simulink model "ampc_pH_lpv"  (R2021a)
settings: Solver=ode45  StartTime=0.0  StopTime=100  MaxStep=0.1  RelTol=1e-3
undefined symbols (not defined in the file or in its folder): sigbuilder_block
libraries: mpclib x1, cstblocks x1, simulink x1
settings Model: Creator=Oluwatofunmi  LastModifiedBy=USER
settings SolverCC: ZeroCrossAlgorithm=Adaptive  AlgebraicLoopSolver=TrustRegion
settings DebuggingCC: PregeneratedLibrarySubsystemCodeDiagnostic=none  SFMachineParentedDataDiag=warning  ArithmeticOperatorsInVariantConditions=warning
settings SFSimCC: CustomCodeUndefinedFunction=UseInterfaceOnly

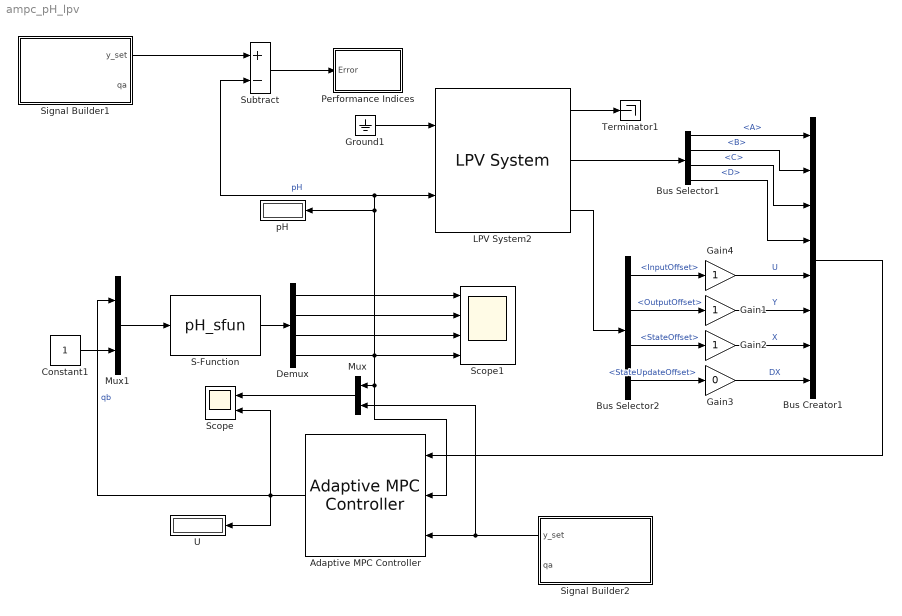
== system ampc_pH_lpv ==
  Adaptive MPC Controller : mpclib/Adaptive MPC Controller  SCDEnableBlockLinearizationSpecification=on  mpcobj=mpcobj_lpv  enable_value=0  updateMPCinCallerWorkspace=on  md_inport=off  mv_inport=off  uref_inport=off  return_cost=off  return_mvseq=off  return_qpstatus=off  return_xseq=off  return_state=off  return_ovseq=off  state_inport=off  isltv_plant=off  umin_inport=off  umax_inport=off  ymin_inport=off  ymax_inport=off  cc_inport=off  ywt_inport=off  uwt_inport=off  duwt_inport=off  rhoeps_inport=off  pm_inport=off  MaximumP=10  HorizonChoice=FixedHorizon  BlockDataType=double  SampleTimeInherited=on  switch_inport=off
  Bus Creator1 : BusCreator  Inputs=8
  Bus Selector1 : BusSelector  OutputSignals=A,B,C,D
  Bus Selector2 : BusSelector  OutputSignals=InputOffset,OutputOffset,StateOffset,StateUpdateOffset
  Constant1 : Constant
  Demux : Demux
  Gain1 : Gain
  Gain2 : Gain
  Gain3 : Gain  Gain=0
  Gain4 : Gain
  Ground1 : Ground
  LPV System2 : cstblocks/Linear Parameter Varying/LPV System  sys=lpv  x0=0  uOffset=lpv_u0  yOffset=lpv_y0  xOffset=lpv_x0  opEquilOption=on  dxOffset=0  sysFixedOption=Use the first model in state-space array  sysFixed=[]  AFixed=false  BFixed=false  CFixed=false  DFixed=false  uDelayFixed=true  yDelayFixed=true  iDelayFixed=true  IMethod=Linear  EMethod=Clip  IndexSearch=Binary search  IndexBegin=on  OutputX=off  OutputXdot=off  OutputLTI=on  OutputOP=on  DataType=double  SimMode=Interpreted execution  InitBufferSize=1024  FixedBuffer=off
      settings: SourceProductBaseCode=CT
  Mux : Mux  Inputs=2
  Mux1 : Mux  Inputs=2
  Performance Indices : Subsystem
  S-Function : S-Function  FunctionName=pH_sfun  SFunctionDeploymentMode=off  EnableBusSupport=off
  Scope : Scope  NumInputPorts=2
  Scope1 : Scope  NumInputPorts=4
  Signal Builder1 : Subsystem  Tag=STV Subsys  LoadFcn=sigbuilder_block('load');  StartFcn=sigbuilder_block('start');  StopFcn=sigbuilder_block('stop');  ClipboardFcn=sigbuilder_block('clipboard');  mask(Sigbuilder block){tuvar=[0:10]}
      mask help: Simulink:masks:SigbuilderBlock_MD
      mask init:
      | if ~strcmp(get_param(bdroot(gcbh),'SimulationStatus'),'stopped') tuvar = sigbuilder_block('maskInit'); end
      settings: CopyFcn=sigbuilder_block('copy');  DeleteFcn=sigbuilder_block('delete');  ModelCloseFcn=sigbuilder_block('modelClose');  PreSaveFcn=sigbuilder_block('preSave');  PauseFcn=sigbuilder_block('pause');  ContinueFcn=sigbuilder_block('continue');  NameChangeFcn=sigbuilder_block('namechange');  OpenFcn=sigbuilder_block('open',[443.25 6 575.25 506.25 ]);  CloseFcn=sigbuilder_block('close');
      mask Display: plot(0, 0, 100, 100,[2, 2, 32, 32, 2], [68, 8, 8, 68, 68],[32, 2], [38, 38], [32, 19, 2],[53, 60, 44], [32, 17, 17, 2],[16, 16, 31, 31]);txt = getActiveGroup(gcbh);text(2, 100, txt,'verticalAlignment', 'top');
  Signal Builder2 : Subsystem  Tag=STV Subsys  LoadFcn=sigbuilder_block('load');  StartFcn=sigbuilder_block('start');  StopFcn=sigbuilder_block('stop');  ClipboardFcn=sigbuilder_block('clipboard');  mask(Sigbuilder block){tuvar=[0:10]}
      mask help: Simulink:masks:SigbuilderBlock_MD
      mask init:
      | if ~strcmp(get_param(bdroot(gcbh),'SimulationStatus'),'stopped') tuvar = sigbuilder_block('maskInit'); end
      settings: CopyFcn=sigbuilder_block('copy');  DeleteFcn=sigbuilder_block('delete');  ModelCloseFcn=sigbuilder_block('modelClose');  PreSaveFcn=sigbuilder_block('preSave');  PauseFcn=sigbuilder_block('pause');  ContinueFcn=sigbuilder_block('continue');  NameChangeFcn=sigbuilder_block('namechange');  OpenFcn=sigbuilder_block('open',[443.25 6 575.25 506.25 ]);  CloseFcn=sigbuilder_block('close');
      mask Display: plot(0, 0, 100, 100,[2, 2, 32, 32, 2], [68, 8, 8, 68, 68],[32, 2], [38, 38], [32, 19, 2],[53, 60, 44], [32, 17, 17, 2],[16, 16, 31, 31]);txt = getActiveGroup(gcbh);text(2, 100, txt,'verticalAlignment', 'top');
  Subtract : Sum  Inputs=+-
  Terminator1 : Terminator
  U : Display
  pH : Display
  wires:
  Ground1/1 -> LPV System2/1
  Bus Selector2/1 -> Gain4/1  "<InputOffset>"
  Gain4/1 -> Bus Creator1/5  "U"
  Bus Selector2/2 -> Gain1/1  "<OutputOffset>"
  Gain1/1 -> Bus Creator1/6  "Y"
  Gain2/1 -> Bus Creator1/7  "X"
  Bus Selector2/3 -> Gain2/1  "<StateOffset>"
  Gain3/1 -> Bus Creator1/8  "DX"
  Bus Selector2/4 -> Gain3/1  "<StateUpdateOffset>"
  Bus Selector1/1 -> Bus Creator1/1  "<A>"
  Bus Selector1/2 -> Bus Creator1/2  "<B>"
  Bus Selector1/3 -> Bus Creator1/3  "<C>"
  Bus Selector1/4 -> Bus Creator1/4  "<D>"
  LPV System2/1 -> Terminator1/1
  Bus Creator1/1 -> Adaptive MPC Controller/1
  Mux/1 -> Scope/1
  Signal Builder2/1(y_set) -> Mux/2, Adaptive MPC Controller/3
  Subtract/1 -> Performance Indices/1(Error)
  Signal Builder1/1(y_set) -> Subtract/1
  Constant1/1 -> Mux1/2
  Mux1/1 -> S-Function/1
  Demux/3 -> Scope1/3
  Demux/2 -> Scope1/2
  Demux/1 -> Scope1/1
  S-Function/1 -> Demux/1
  Demux/4 -> Adaptive MPC Controller/2, Mux/1, Scope1/4, LPV System2/2, Subtract/2, pH/1  "pH"
  Adaptive MPC Controller/1 -> Mux1/1, U/1, Scope/2  "qb"
  LPV System2/3 -> Bus Selector2/1
  LPV System2/2 -> Bus Selector1/1

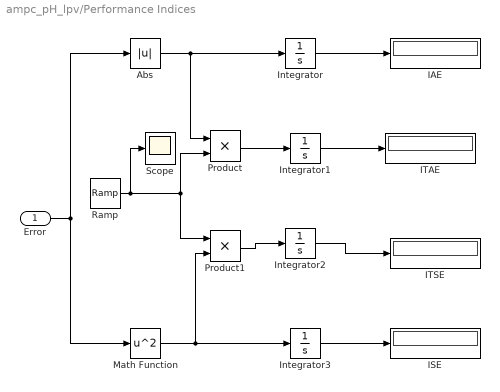
== system ampc_pH_lpv/Performance Indices ==
  Error : Inport
  Abs : Abs
  IAE : Display
  ISE : Display
  ITAE : Display
  ITSE : Display
  Integrator{,1..3} (4 alike) : Integrator
  Math Function : Math  Operator=square  SignedPower=on  SaturateOnIntegerOverflow=on
  Product : Product  RndMeth=Zero
  Product1 : Product  RndMeth=Zero
  Ramp : simulink/Sources/Ramp  slope=1  start=0  InitialOutput=0
  Scope : Scope
  wires:
  Error/1 -> Math Function/1, Abs/1
  Abs/1 -> Integrator/1, Product/1
  Integrator/1 -> IAE/1
  Ramp/1 -> Product/2, Product1/1, Scope/1
  Math Function/1 -> Integrator3/1, Product1/2
  Product1/1 -> Integrator2/1
  Product/1 -> Integrator1/1
  Integrator3/1 -> ISE/1
  Integrator2/1 -> ITSE/1
  Integrator1/1 -> ITAE/1

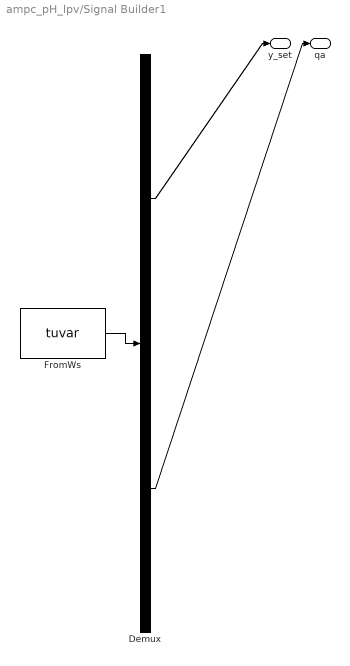
== system ampc_pH_lpv/Signal Builder1 ==
  Demux : Demux  Tag=STV Demux  Outputs=2
      settings: DisplayOption=none
  FromWs : FromWorkspace  Tag=STV FromWs  VariableName=tuvar
      SigBuilderData=|
      | common.afterFinalStr = 'Extrapolate'
      | common.sampleTime = 0
      | dataSet(1).timeRange = [0 100]
      | dataSet(1).name = 'Servo'
      | dataSet(2).timeRange = [0 70]
      | dataSet(2).name = 'Regulatory'
      | sbobj.Groups(1).Name = 'Servo'
      | sbobj.Groups(1).Signals(1).Name = 'y_set'
      | sbobj.Groups(1).Signals(1).XData = [0 10 10 20 20 30 30 40 40 50 50 60 60 70 70 100]
      | sbobj.Groups(1).Signals(1).YData = [3.14776 3.14776 5 5 6 6 7 7 8 8 9 9 10 10 5 5]
      | sbobj.Groups(1).Signals(2).Name = 'qa'
      | sbobj.Groups(1).Signals(2).XData = [0 100]
      | sbobj.Groups(1).Signals(2).YData = [1 1]
      | sbobj.Groups(1).TimeRange = [0 100]
      | sbobj.Groups(2).Name = 'Regulatory'
      | sbobj.Groups(2).Signals(1).Name = 'y_set'
      | sbobj.Groups(2).Signals(1).XData = [0 70]
      | sbobj.Groups(2).Signals(1).YData = [7.01 7.01]
      | sbobj.Groups(2).Signals(2).Name = 'qa'
      | sbobj.Groups(2).Signals(2).XData = [0 10 10 20 20 30 30 40 40 50 50 70]
      | sbobj.Groups(2).Signals(2).YData = [1 1 1.5 1.5 1 1 0.5 0.5 1.5 1.5 1 1]
      | sbobj.Groups(2).TimeRange = [0 70]
  y_set : Outport  Tag=STV Outport  VectorParamsAs1DForOutWhenUnconnected=off
  qa : Outport  Tag=STV Outport  Port=2  VectorParamsAs1DForOutWhenUnconnected=off
  wires:
  FromWs/1 -> Demux/1
  Demux/1 -> y_set/1
  Demux/2 -> qa/1

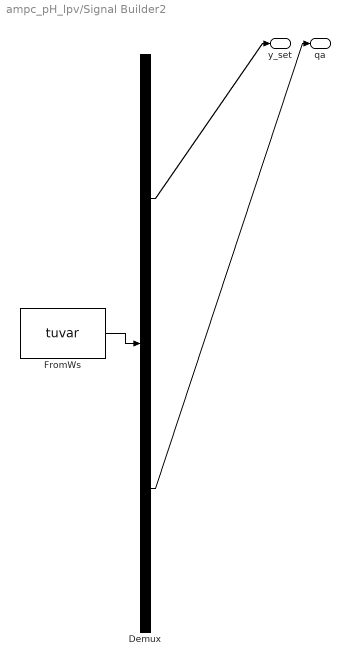
== system ampc_pH_lpv/Signal Builder2 ==
  Demux : Demux  Tag=STV Demux  Outputs=2
      settings: DisplayOption=none
  FromWs : FromWorkspace  Tag=STV FromWs  VariableName=tuvar
      SigBuilderData=|
      | common.afterFinalStr = 'Extrapolate'
      | common.sampleTime = 0
      | dataSet(1).timeRange = [0 100]
      | dataSet(1).name = 'Servo'
      | dataSet(2).timeRange = [0 70]
      | dataSet(2).name = 'Regulatory'
      | sbobj.Groups(1).Name = 'Servo'
      | sbobj.Groups(1).Signals(1).Name = 'y_set'
      | sbobj.Groups(1).Signals(1).XData = [0 10 10 20 20 30 30 40 40 50 50 60 60 70 70 100]
      | sbobj.Groups(1).Signals(1).YData = [3.14776 3.14776 5 5 6 6 7 7 8 8 9 9 10 10 5 5]
      | sbobj.Groups(1).Signals(2).Name = 'qa'
      | sbobj.Groups(1).Signals(2).XData = [0 100]
      | sbobj.Groups(1).Signals(2).YData = [1 1]
      | sbobj.Groups(1).TimeRange = [0 100]
      | sbobj.Groups(2).Name = 'Regulatory'
      | sbobj.Groups(2).Signals(1).Name = 'y_set'
      | sbobj.Groups(2).Signals(1).XData = [0 70]
      | sbobj.Groups(2).Signals(1).YData = [7.01 7.01]
      | sbobj.Groups(2).Signals(2).Name = 'qa'
      | sbobj.Groups(2).Signals(2).XData = [0 10 10 20 20 30 30 40 40 50 50 70]
      | sbobj.Groups(2).Signals(2).YData = [1 1 1.5 1.5 1 1 0.5 0.5 1.5 1.5 1 1]
      | sbobj.Groups(2).TimeRange = [0 70]
  y_set : Outport  Tag=STV Outport  VectorParamsAs1DForOutWhenUnconnected=off
  qa : Outport  Tag=STV Outport  Port=2  VectorParamsAs1DForOutWhenUnconnected=off
  wires:
  FromWs/1 -> Demux/1
  Demux/1 -> y_set/1
  Demux/2 -> qa/1
